simulink model "aircraft_controls"  (R2015b)
settings: Solver=ode45  StartTime=0.0  StopTime=10000  RelTol=1e-3
values from neighbouring files (symbols this model uses):
  control_surfaces_constant = control_surfaces0    [RunSimLab6.m]
  delta_deltae = stuff(2)    [unknown_vars.m]
  DRAW_FLAG = 0    [RunSimLab6.m]
  wind_inertial = [0;0;0]    [RunSimLab6.m]
undefined symbols (not defined in the file or in its folder): aircraft_parameters, drawAircraft, PlotStateVariables, pts, S_AeroForcesAndMoments
libraries: aerolibobsolete x1, aerolibatmos2 x1
settings Model: Creator=beard  LastModifiedBy=Jeremy
settings DataIOCC: SaveFormat=Array  SignalLoggingSaveFormat=ModelDataLogs
settings OptimizationCC: ExpressionDepthLimit=2147483647  InitFltsAndDblsToZero=on
settings DebuggingCC: UnderspecifiedInitializationDetection=Classic  MergeDetectMultiDrivingBlocksExec=none  SolverPrmCheckMsg=warning  FcnCallInpInsideContextMsg=UseLocalSettings  StateNameClashWarn=warning
settings HardwareCC: ProdBitPerPointer=32  ProdLargestAtomicFloat=None  ProdIntDivRoundTo=Undefined  ProdEndianess=Unspecified  ProdWordSize=32  ProdHWDeviceType=32-bit Generic
settings GRTTargetCC: GeneratePreprocessorConditionals=Disable all  CombineOutputUpdateFcns=off  GRTInterface=on
settings ConfigComp: CovModelRefEnable=Off  CovSFcnEnable=off

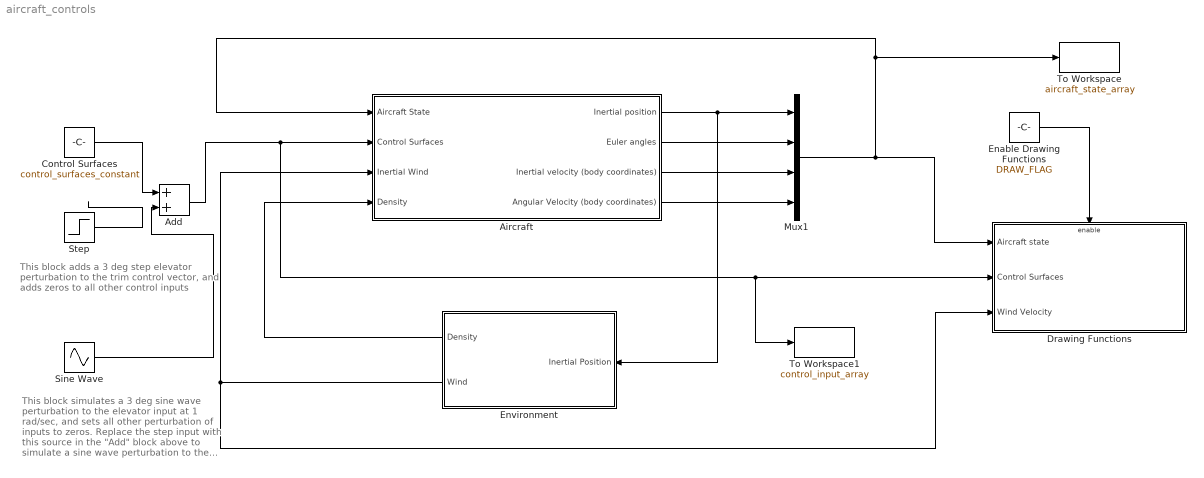
== system aircraft_controls ==
  note: This block simulates a 3 deg sine
      | wave perturbation to the elevator
      | input at 1 rad/sec, and sets all other
      | perturbation of inputs to zeros.
      | Replace the step input with this source
      | in the "Add" block above to simulate
      | a sine wave perturbation to the control
      | inputs about the trim conditions.
  note: This block adds a 3 deg step elevator
      | perturbation to the trim control vector,
      | and adds zeros to all other control inputs
  Add : Sum
  Aircraft : Subsystem
  Control Surfaces : Constant  Value=control_surfaces_constant
  Drawing Functions : Subsystem  TreatAsAtomicUnit=on
  Enable Drawing Functions : Constant  Value=DRAW_FLAG
  Environment : Subsystem
  Mux1 : Mux
  Sine Wave : Sin  Amplitude=[5*pi/180 ;0 ; 0 ; 0]  Bias=[0;0;0;0];  Frequency=0.536114500304593/10  SampleTime=0  VectorParams1D=off
  Step : Step  Before=[0;0;0;0]  After=[delta_deltae;0;0;0]  SampleTime=0  VectorParams1D=off
  To Workspace : ToWorkspace  VariableName=aircraft_state_array  SaveFormat=Timeseries  SampleTime=-1
  To Workspace1 : ToWorkspace  VariableName=control_input_array  SaveFormat=Timeseries  SampleTime=-1
  wires:
  Mux1/1 -> Drawing Functions/1(Aircraft state), Aircraft/1(Aircraft State), To Workspace/1
  Environment/1(Density) -> Aircraft/4(Density)
  Environment/2(Wind) -> Drawing Functions/3(Wind Velocity), Aircraft/3(Inertial Wind)
  Aircraft/4(Angular Velocity (body coordinates)) -> Mux1/4
  Aircraft/3(Inertial velocity (body coordinates)) -> Mux1/3
  Aircraft/2(Euler angles) -> Mux1/2
  Aircraft/1(Inertial position) -> Mux1/1, Environment/1(Inertial Position)
  Enable Drawing Functions/1 -> Drawing Functions/Enable
  Step/1 -> ?
  Control Surfaces/1 -> Add/1
  Add/1 -> Drawing Functions/2(Control Surfaces), To Workspace1/1, Aircraft/2(Control Surfaces)
  Sine Wave/1 -> Add/2

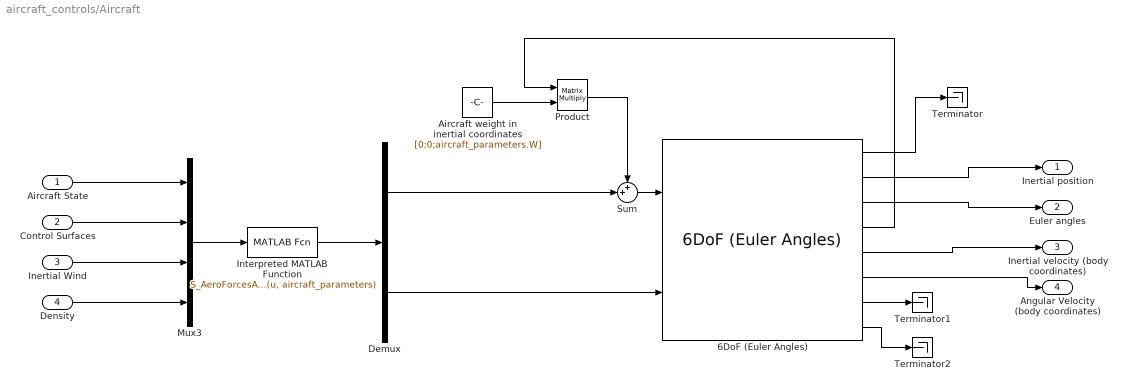
== system aircraft_controls/Aircraft ==
  Aircraft State : Inport
  Control Surfaces : Inport  Port=2
  Inertial Wind : Inport  Port=3
  Density : Inport  Port=4
  6DoF (Euler Angles) : aerolibobsolete/6DoF (Euler Angles)  units=Metric (MKS)  mtype=Fixed  rep=Euler Angles  xme_0=position_inertial  Vm_0=velocity_body  eul_0=euler_angles  pm_0=omega_body  mass_0=aircraft_parameters.m  mass_e=0.5  mass_f=2.0  inertia=inertia_matrix  inertia_e=eye(3)  inertia_f=2*eye(3)  k_quat=1.0
  Aircraft weight in inertial coordinates : Constant  Value=[0;0;aircraft_parameters.W]
  Demux : Demux  Outputs=2
  Interpreted MATLAB Function : MATLABFcn  MATLABFcn=S_AeroForcesAndMoments(u, aircraft_parameters)  OutputDimensions=6
  Mux3 : Mux
  Product : Product  Multiplication=Matrix(*)  RndMeth=Zero
  Sum : Sum  Inputs=++|
  Terminator : Terminator
  Terminator1 : Terminator
  Terminator2 : Terminator
  Inertial position : Outport
  Euler angles : Outport  Port=2
  Inertial velocity (body coordinates) : Outport  Port=3
  Angular Velocity (body coordinates) : Outport  Port=4
  wires:
  6DoF (Euler Angles)/2 -> Inertial position/1
  6DoF (Euler Angles)/3 -> Euler angles/1
  6DoF (Euler Angles)/5 -> Inertial velocity (body coordinates)/1
  6DoF (Euler Angles)/6 -> Angular Velocity (body coordinates)/1
  6DoF (Euler Angles)/4 -> Product/1
  Sum/1 -> 6DoF (Euler Angles)/1
  Product/1 -> Sum/1
  Aircraft weight in inertial coordinates/1 -> Product/2
  Mux3/1 -> Interpreted MATLAB Function/1
  Demux/1 -> Sum/2
  Demux/2 -> 6DoF (Euler Angles)/2
  Interpreted MATLAB Function/1 -> Demux/1
  Control Surfaces/1 -> Mux3/2
  6DoF (Euler Angles)/1 -> Terminator/1
  6DoF (Euler Angles)/7 -> Terminator1/1
  6DoF (Euler Angles)/8 -> Terminator2/1
  Aircraft State/1 -> Mux3/1
  Inertial Wind/1 -> Mux3/3
  Density/1 -> Mux3/4

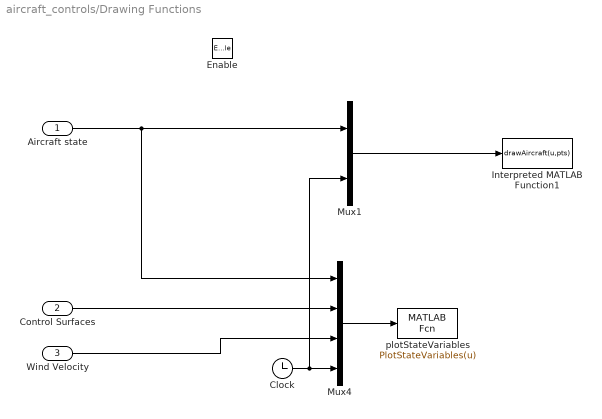
== system aircraft_controls/Drawing Functions ==
  Aircraft state : Inport
  Control Surfaces : Inport  Port=2
  Wind Velocity : Inport  Port=3
  Enable : EnablePort
  Clock : Clock
  Interpreted MATLAB Function1 : MATLABFcn  MATLABFcn=drawAircraft(u,pts)  OutputDimensions=0
  Mux1 : Mux  Inputs=2
  Mux4 : Mux
  plotStateVariables : MATLABFcn  MATLABFcn=PlotStateVariables(u)  OutputDimensions=0  SampleTime=.1
  wires:
  Mux4/1 -> plotStateVariables/1
  Control Surfaces/1 -> Mux4/2
  Wind Velocity/1 -> Mux4/3
  Clock/1 -> Mux1/2, Mux4/4
  Aircraft state/1 -> Mux1/1, Mux4/1
  Mux1/1 -> Interpreted MATLAB Function1/1

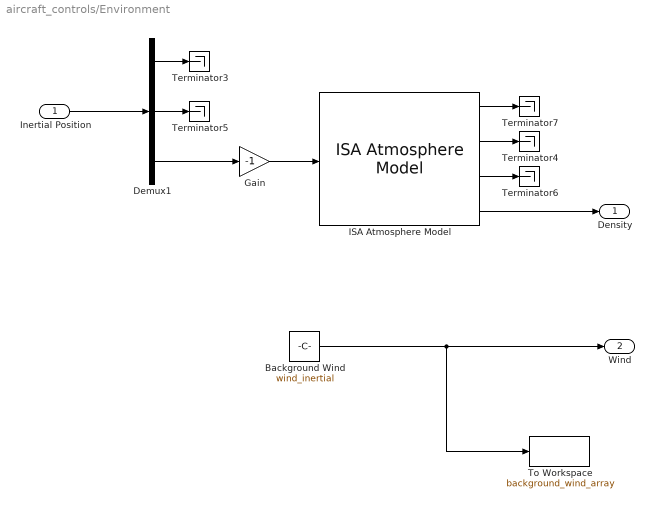
== system aircraft_controls/Environment ==
  Inertial Position : Inport
  Background Wind : Constant  Value=wind_inertial
  Demux1 : Demux  Outputs=3
  Gain : Gain  Gain=-1
  ISA Atmosphere Model : aerolibatmos2/ISA Atmosphere Model  custom=off  g=9.80665  gamma=1.4  R=287.0531  L=0.0065  h_trop=11000  h_strat=20000  rho0=1.225  P0=101325  T0=288.15  h0=0
  Terminator{3..7} (5 alike) : Terminator
  To Workspace : ToWorkspace  VariableName=background_wind_array  SaveFormat=Timeseries  SampleTime=-1
  Density : Outport
  Wind : Outport  Port=2
  wires:
  Inertial Position/1 -> Demux1/1
  Demux1/3 -> Gain/1
  Gain/1 -> ISA Atmosphere Model/1
  Demux1/1 -> Terminator3/1
  Demux1/2 -> Terminator5/1
  ISA Atmosphere Model/3 -> Terminator6/1
  ISA Atmosphere Model/2 -> Terminator4/1
  ISA Atmosphere Model/1 -> Terminator7/1
  ISA Atmosphere Model/4 -> Density/1
  Background Wind/1 -> To Workspace/1, Wind/1
